simulink model "wiper_mechanism_signal_builder"  (R2020a)
settings: Solver=FixedStepDiscrete  StartTime=0.0  StopTime=0.5  FixedStep=0.1  RelTol=1e-3
undefined symbols (not defined in the file or in its folder): sigbuilder_block
settings Model: Creator=Kundan Patil  LastModifiedBy=Kundan Patil

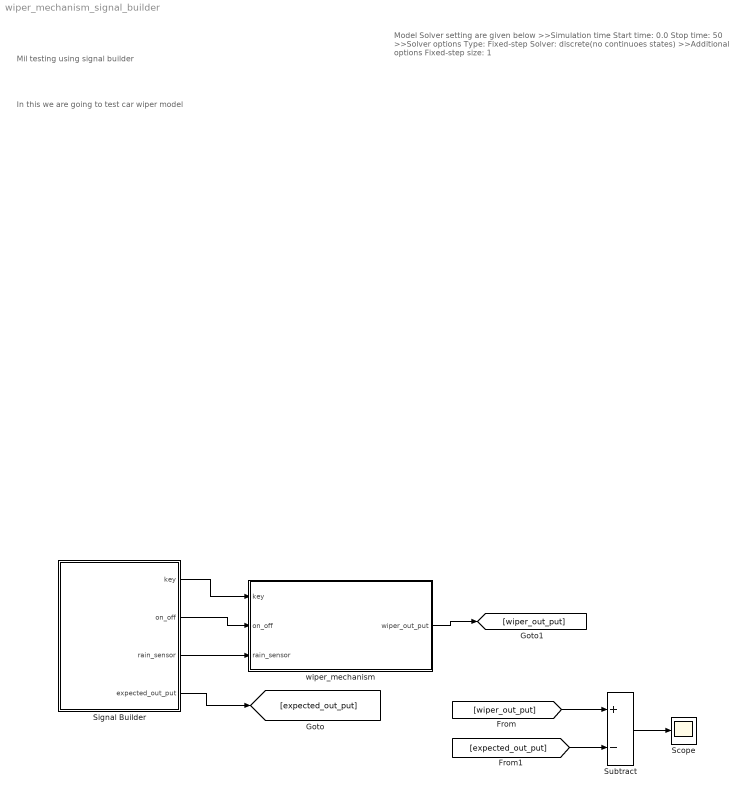
== system wiper_mechanism_signal_builder ==
  note: Model Solver setting are given below
      | >>Simulation time
      | 		Start time: 0.0
      | 		Stop time: 50
      | >>Solver options
      | 		Type: Fixed-step
      | 		Solver: discrete(no continuoes states)
      | >>Additional options
      | 		Fixed-step size: 1
  note: In this we are going to test car wiper model
  note: Mil testing using signal builder
  Scope : Scope
  Signal Builder : Subsystem  Tag=STV Subsys  LoadFcn=sigbuilder_block('load');  StartFcn=sigbuilder_block('start');  StopFcn=sigbuilder_block('stop');  ClipboardFcn=sigbuilder_block('clipboard');  mask(Sigbuilder block){tuvar=[0:10]}
      mask help: Simulink:masks:SigbuilderBlock_MD
      mask init:
      | if ~strcmp(get_param(bdroot(gcbh),'SimulationStatus'),'stopped') tuvar = sigbuilder_block('maskInit'); end
      settings: CopyFcn=sigbuilder_block('copy');  DeleteFcn=sigbuilder_block('delete');  ModelCloseFcn=sigbuilder_block('modelClose');  PreSaveFcn=sigbuilder_block('preSave');  PauseFcn=sigbuilder_block('pause');  ContinueFcn=sigbuilder_block('continue');  NameChangeFcn=sigbuilder_block('namechange');  OpenFcn=sigbuilder_block('open',[438.6 158.4 550.8 400.2 ]);  CloseFcn=sigbuilder_block('close');
      mask Display: plot(0, 0, 100, 100,[2, 2, 32, 32, 2], [68, 8, 8, 68, 68],[32, 2], [38, 38], [32, 19, 2],[53, 60, 44], [32, 17, 17, 2],[16, 16, 31, 31]);txt = getActiveGroup(gcbh);text(2, 100, txt,'verticalAlignment', 'top');
  Subtract : Sum  Inputs=+-
  wiper_mechanism : Subsystem
  wires:
  Signal Builder/1(key) -> wiper_mechanism/1(key)
  Signal Builder/2(on_off) -> wiper_mechanism/2(on_off)
  Signal Builder/3(rain_sensor) -> wiper_mechanism/3(rain_sensor)
  Signal Builder/4(expected_out_put) -> [expected_out_put]
  wiper_mechanism/1(wiper_out_put) -> [wiper_out_put]
  [wiper_out_put] -> Subtract/1
  [expected_out_put] -> Subtract/2
  Subtract/1 -> Scope/1

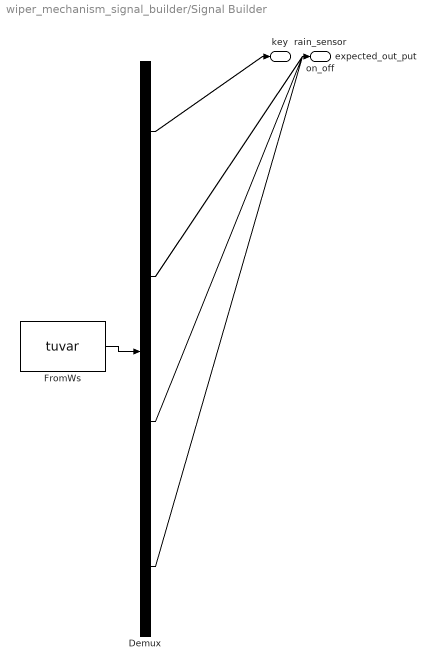
== system wiper_mechanism_signal_builder/Signal Builder ==
  Demux : Demux  Tag=STV Demux
      settings: DisplayOption=none
  FromWs : FromWorkspace  Tag=STV FromWs  VariableName=tuvar
      SigBuilderData=|
      | common.afterFinalStr = 'Extrapolate'
      | common.sampleTime = 0
      | dataSet.timeRange = [0 0.5]
      | dataSet.name = 'Group 1'
      | sbobj.Groups.Name = 'Group 1'
      | sbobj.Groups.Signals(1).Name = 'key'
      | sbobj.Groups.Signals(1).XData = [0 0.1 0.1 0.2 0.3 0.4 0.5]
      | sbobj.Groups.Signals(1).YData = [0 0 1 1 1 1 1]
      | sbobj.Groups.Signals(2).Name = 'on_off'
      | sbobj.Groups.Signals(2).XData = [0 0.1 0.1 0.2 0.2 0.3 0.3 0.4 0.4 0.5]
      | sbobj.Groups.Signals(2).YData = [0 0 1 1 -0.02 0 1 1 0 0]
      | sbobj.Groups.Signals(3).Name = 'rain_sensor'
      | sbobj.Groups.Signals(3).XData = [0 0.1 0.2 0.2 0.3 0.4 0.4 0.5]
      | sbobj.Groups.Signals(3).YData = [0 0 0 1 1 1 0 0]
      | sbobj.Groups.Signals(4).Name = 'expected_out_put'
      | sbobj.Groups.Signals(4).XData = [0 0.1 0.1 0.3 0.4 0.4 0.5]
      | sbobj.Groups.Signals(4).YData = [0 0 1 1 1 0 0]
      | sbobj.Groups.TimeRange = [0 0.5]
  key : Outport  Tag=STV Outport
  on_off : Outport  Tag=STV Outport  Port=2
  rain_sensor : Outport  Tag=STV Outport  Port=3
  expected_out_put : Outport  Tag=STV Outport  Port=4
  wires:
  FromWs/1 -> Demux/1
  Demux/1 -> key/1
  Demux/2 -> on_off/1
  Demux/3 -> rain_sensor/1
  Demux/4 -> expected_out_put/1

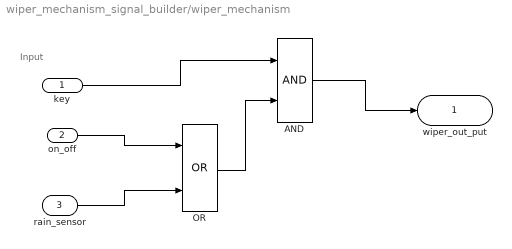
== system wiper_mechanism_signal_builder/wiper_mechanism ==
  note: Input
  key : Inport
  on_off : Inport  Port=2
  rain_sensor : Inport  Port=3
  AND : Logic  AllPortsSameDT=off  OutDataTypeStr=boolean
  OR : Logic  Operator=OR  AllPortsSameDT=off  OutDataTypeStr=boolean
  wiper_out_put : Outport
  wires:
  on_off/1 -> OR/1
  AND/1 -> wiper_out_put/1
  rain_sensor/1 -> OR/2
  OR/1 -> AND/2
  key/1 -> AND/1
